simulink model "mariner_sim"  (R2018b)
settings: Solver=VariableStepAuto  StartTime=0.0  StopTime=10  RelTol=1e-3
libraries: simulink x1
settings Model: Creator=manzand  LastModifiedBy=manzand

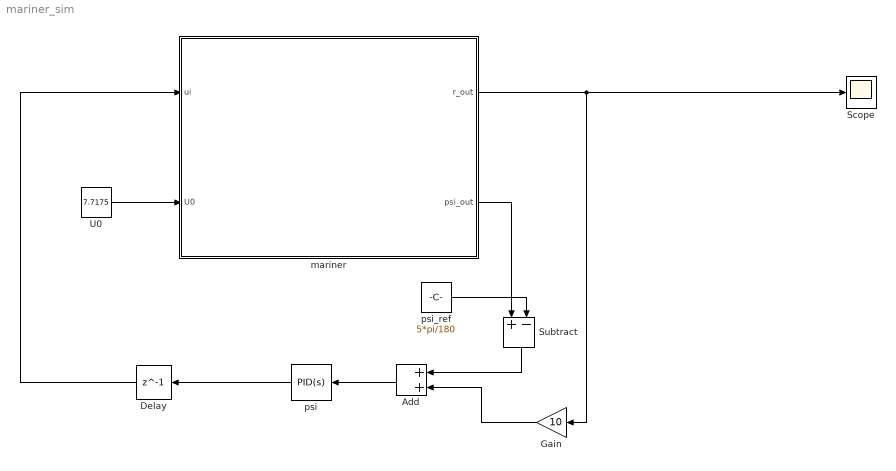
== system mariner_sim ==
  Add : Sum
  Delay : Delay  DelayLength=1  InitialCondition=0
  Gain : Gain  Gain=10
  Scope : Scope
  Subtract : Sum  Inputs=+-
  U0 : Constant  Value=7.7175
  mariner : Stateflow chart  TreatAsAtomicUnit=on
  psi : simulink/Continuous/PID Controller  Controller=PID  Form=Parallel  TimeDomain=Continuous-time  SampleTime=-1  IntegratorMethod=Forward Euler  FilterMethod=Forward Euler  ControllerParametersSource=internal  P=-1  I=0  D=0  UseFilter=on  N=100  TunerSelectOption=Transfer Function Based (PID Tuner App)  InitialConditionSource=internal  InitialConditionForIntegrator=0  InitialConditionForFilter=0  DifferentiatorICPrevScaledInput=0  ExternalReset=none  TrackingMode=off  Kt=1  LimitOutput=off  UpperSaturationLimit=inf  LowerSaturationLimit=-inf  LinearizeAsGain=on  AntiWindupMode=none  Kb=1  POutMin=[]  POutMax=[]  IOutMin=[]  IOutMax=[]  DOutMin=[]  DOutMax=[]  NOutMin=[]  NOutMax=[]  SumOutMin=[]  SumOutMax=[]  SaturationOutMin=[]  SaturationOutMax=[]  PParamMin=[]  PParamMax=[]  IParamMin=[]  IParamMax=[]  DParamMin=[]  DParamMax=[]  NParamMin=[]  NParamMax=[]  KbParamMin=[]  KbParamMax=[]  KtParamMin=[]  KtParamMax=[]  KbOutMin=[]  KbOutMax=[]  KtOutMin=[]  KtOutMax=[]  IntegratorOutMin=[]  IntegratorOutMax=[]  FilterOutMin=[]  FilterOutMax=[]  SumI1OutMin=[]  SumI1OutMax=[]  SumI2OutMin=[]  SumI2OutMax=[]  SumI3OutMin=[]  SumI3OutMax=[]  SumI4OutMin=[]  SumI4OutMax=[]  SumDOutMin=[]  SumDOutMax=[]  DifferentiatorOutMin=[]  DifferentiatorOutMax=[]  FilterDiffOutCoefMin=[]  FilterDiffOutCoefMax=[]  ReciprocalOutMin=[]  ReciprocalOutMax=[]  SumDenOutMin=[]  SumDenOutMax=[]  SumNumOutMin=[]  SumNumOutMax=[]  DivideOutMin=[]  DivideOutMax=[]  IntegratorContinuousStateAttributes=''  IntegratorStateMustResolveToSignalObject=off  IntegratorRTWStateStorageClass=Auto  FilterContinuousStateAttributes=''  FilterStateMustResolveToSignalObject=off  FilterRTWStateStorageClass=Auto  ParallelPVariant=InternalParameters  IdealPVariant=Disabled  IVariant=InternalParameters  DVariant=InternalParameters  IntegratorVariant=Continuous  SatVariant=Disabled  AWVariant=Passthrough  PCopyVariant=Disabled  TRVariant=Disabled  FdbkBlocksVariant=Forward  IdealPFdbkVariant=Disabled  SatFdbkVariant=Disabled  DerivativeFilterVariant=ContFilter  NVariant=InternalParameters  NCopyVariant=Disabled  FilterICVariant=InternalICsFilter  IntegratorICVariant=InternalICs  ExternalResetVariant=Disabled  TRSumVariant=Passthrough  SumFdbkVariant=Disabled  SumVariant=Sum_PID
  psi_ref : Constant  Value=5*pi/180
  wires:
  U0/1 -> mariner/2(U0)
  mariner/1(r_out) -> Scope/1, Gain/1
  mariner/2(psi_out) -> Subtract/1
  psi_ref/1 -> Subtract/2
  Subtract/1 -> Add/1
  Gain/1 -> Add/2
  Add/1 -> psi/1
  psi/1 -> Delay/1
  Delay/1 -> mariner/1(ui)

== stateflow chart mariner_sim/mariner ==
  settings: updateMethod=CONTINUOUS
  state mariner
    %% initialize values when entry
    en:
    L = 160.93;
    m = 798*10^-5;
    xG = -0.023;
    Iz = 39.2*10^-5;
    Xudot =  -42e-5;  Yvdot =  -748e-5;  Nvdot = 4.646e-5;
    Xu  = -184e-5;   Yrdot =-9.354e-5;   Nrdot = -43.8e-5;
    Xuu = -110e-5;   Yv = -1160e-5;   Nv =  -264e-5;
    Xuuu = -215e-5;   Yr =  -499e-5;   Nr =  -166e-5;
    Xvv = -899e-5;   Yvvv = -8078e-5;   Nvvv =  1636e-5;
    Xrr =   18e-5;   Yvvr = 15356e-5;   Nvvr = -5483e-5;
    Xdd =  -95e-5;   Yvu = -1160e-5;   Nvu =  -264e-5;
    Xudd = -190e-5;   Yru =  -499e-5;   Nru =  -166e-5;
    Xrv =  798e-5;   Yd  =   278e-5;   Nd =  -139e-5;
    Xvd =   93e-5;   Yddd  =   -90e-5;   Nddd =    45e-5;
    Xuvd =   93e-5;   Yud = 556e-5;   Nud =  -278e-5;
    Yuud =   278e-5;   Nuud  =  -139e-5;
    Yvdd  =    -4e-5;   Nvdd  = 13e-5;
    Yvvd  =  1190e-5;   Nvvd  = -489e-5;
    Y0 = -4e-5;   N0 =  3e-5;
    Y0u  =  -8e-5;   N0u = 6e-5;
    Y0uu =  -4e-5;   N0uu  =  3e-5;
    m11 = 798*10^-5 - (-42e-5);
    m22 = 798*10^-5 - ( -748e-5);
    m23 = 798*10^-5 * -0.023 - (-9.354e-5);
    m32 = 798*10^-5 * -0.023 - 4.646e-5;
    m33 = 39.2*10^-5 -  (-43.8e-5);
    %detM22 = m22*m33-m23*m32;
    %detM22 = ((798*10^-5 - ( -748e-5))*(39.2*10^-5 -  (-43.8e-5)) - (798*10^-5 * -0.023 - (-9.354e-5))*(798*10^-5 * -0.023 - 4.646e-5));
    delta_max = 40;
    Ddelta_max = 5;
    % u
    %Executing updates of system during simulation
    du:
    %delta_c = min(max(-ui,-delta_max*pi/180),delta_max*pi/180) ;
    %U = (sqrt((ui + u)^2 + v^2));
    %delta_do = (-ui - delta);
    %X = Xu*u/(sqrt((ui + u)^2 + v^2)) + Xuu*(u/(sqrt((ui + u)^2 + v^2)))^2 + Xuuu*(u/(sqrt((ui + u)^2 + v^2)))^3 + Xvv*(v/(sqrt((ui + u)^2 + v^2)))^2 + Xrr*(r*L/(sqrt((ui + u)^2 + v^2)))^2 + Xrv*(r*L/(sqrt((ui + u)^2 + v^2)))*(v/(sqrt((ui + u)^2 + v^2))) + Xdd*delta^2 +Xudd*(u/(sqrt((ui + u)^2 + v^2)))*delta^2 + Xvd*(v/(sqrt((ui + u)^2 + v^2)))*delta + Xuvd*(u/(sqrt((ui + u)^2 + v^2)))*(v/(sqrt((ui + u)^2 + v^2)))*delta;
    %Y = Yv*v + Yr*r + Yvvv*v^3 + Yvvr*v^2*r + Yvu*v*u + Yru*r*u + Yd*delta + Yddd*delta^3 + Yud*u*delta + Yuud*u^2*delta + Yvdd*v*delta^2 + Yvvd*v^2*delta + (Y0 + Y0u*u + Y0uu*u^2);
    %N = Nv*v + Nr*r + Nvvv*v^3 + Nvvr*v^2*r + Nvu*v*u + Nru*r*u + Nd*delta + Nddd*delta^3 + Nud*u*delta + Nuud*u^2*delta + Nvdd*v*delta^2 + Nvvd*v^2*delta + (N0 + N0u*u + N0uu*u^2);
    u_dot = (Xu*(u/(sqrt((ui + u)^2 + v^2))) + Xuu*(u/(sqrt((ui + u)^2 + v^2)))^2 + Xuuu*(u/(sqrt((ui + u)^2 + v^2)))^3 + Xvv*(v/(sqrt((ui + u)^2 + v^2)))^2 + Xrr*(r*L/(sqrt((ui + u)^2 + v^2)))^2 + Xrv*(r*L/(sqrt((ui + u)^2 + v^2)))*(v/(sqrt((ui + u)^2 + v^2))) + Xdd*delta^2 +Xudd*(u/(sqrt((ui + u)^2 + v^2)))*delta^2 + Xvd*(v/(sqrt((ui + u)^2 + v^2)))*delta + Xuvd*(u/(sqrt((ui + u)^2 + v^2)))*(v/(sqrt((ui + u)^2 + v^2)))*delta)*((sqrt((ui + u)^2 + v^2))^2 /L)/(798*10^-5 - (-42e-5));
    v_dot =  -(-(39.2*10^-5 -  (-43.8e-5))*(Yv*(v/(sqrt((ui + u)^2 + v^2))) + Yr*(r*L/(sqrt((ui + u)^2 + v^2))) + Yvvv*(v/(sqrt((ui + u)^2 + v^2)))^3 + Yvvr*(v/(sqrt((ui + u)^2 + v^2)))^2 * (r*L/(sqrt((ui + u)^2 + v^2))) + Yvu*(v/(sqrt((ui + u)^2 + v^2)))*(u/(sqrt((ui + u)^2 + v^2))) + Yru*(r*L/(sqrt((ui + u)^2 + v^2)))*(u/(sqrt((ui + u)^2 + v^2))) + Yd*delta + Yddd*delta^3 + Yud*(u/(sqrt((ui + u)^2 + v^2)))*delta + Yuud*(u/(sqrt((ui + u)^2 + v^2)))^2*delta + Yvdd*(v/(sqrt((ui + u)^2 + v^2)))*delta^2 + Yvvd*(v/(sqrt((ui + u)^2 + v^2)))^2*delta + (Y0 + Y0u*(u/(sqrt((ui + u)^2 + v^2))) + Y0uu*(u/(sqrt((ui + u)^2 + v^2)))^2))+(798*10^-5 * -0.023 - (-9.354e-5))*(Nv*(v/(sqrt((ui + u)^2 + v^2))) + Nr*(r*L/(sqrt((ui + u)^2 + v^2))) + Nvvv*(v/(sqrt((ui + u)^2 + v^2)))^3 + Nvvr*(v/(sqrt((ui + u)^2 + v^2)))^2*(r*L/(sqrt((ui + u)^2 + v^2))) + Nvu*(v/(sqrt((ui + u)^2 + v^2)))*(u/(sqrt((ui + u)^2 + v^2))) + Nru*(r*L/(sqrt((ui + u)^2 + v^2)))*(u/(sqrt((ui + u)^2 + v^2))) + Nd*delta + Nddd*delta^3 + Nud*(u/(sqrt((ui + u)^2 + v^2)))*delta + Nuud*(u/(sqrt((ui + u)^2 + v^2)))^2*delta + Nvdd*(v/(sqrt((ui + u)^2 + v^2)))*delta^2 + Nvvd*v^2*delta + (N0 + N0u*u + N0uu*u^2)))*((sqrt((ui + u)^2 + v^2))^2/L)/((798*10^-5 - ( -748e-5))*(39.2*10^-5 -  (-43.8e-5)) - (798*10^-5 * -0.023 - (-9.354e-5))*(798*10^-5 * -0.023 - 4.646e-5)) ;
    r_dot = (-(798*10^-5 * -0.023 - 4.646e-5)*(Yv*(v/(sqrt((ui + u)^2 + v^2))) + Yr*(r*L/(sqrt((ui + u)^2 + v^2))) + Yvvv*(v/(sqrt((ui + u)^2 + v^2)))^3 + Yvvr*(v/(sqrt((ui + u)^2 + v^2)))^2*(r*L/(sqrt((ui + u)^2 + v^2))) + Yvu*(v/(sqrt((ui + u)^2 + v^2)))*(u/(sqrt((ui + u)^2 + v^2))) + Yru*(r*L/(sqrt((ui + u)^2 + v^2)))*(u/(sqrt((ui + u)^2 + v^2))) + Yd*delta + Yddd*delta^3 + Yud*(u/(sqrt((ui + u)^2 + v^2)))*delta + Yuud*(u/(sqrt((ui + u)^2 + v^2)))^2*delta + Yvdd*(v/(sqrt((ui + u)^2 + v^2)))*delta^2 + Yvvd*(v/(sqrt((ui + u)^2 + v^2)))^2*delta + (Y0 + Y0u*(u/(sqrt((ui + u)^2 + v^2))) + Y0uu*(u/(sqrt((ui + u)^2 + v^2)))^2))+(798*10^-5 - ( -748e-5))*(Nv*(v/(sqrt((ui + u)^2 + v^2))) + Nr*(r*L/(sqrt((ui + u)^2 + v^2))) + Nvvv*(v/(sqrt((ui + u)^2 + v^2)))^3 + Nvvr*(v/(sqrt((ui + u)^2 + v^2)))^2*(r*L/(sqrt((ui + u)^2 + v^2))) + Nvu*(v/(sqrt((ui + u)^2 + v^2)))*(u/(sqrt((ui + u)^2 + v^2))) + Nru*(r*L/(sqrt((ui + u)^2 + v^2)))*(u/(sqrt((ui + u)^2 + v^2))) + Nd*delta + Nddd*delta^3 + Nud*(u/(sqrt((ui + u)^2 + v^2)))*delta + Nuud*(u/(sqrt((ui + u)^2 + v^2)))^2*delta + Nvdd*(v/(sqrt((ui + u)^2 + v^2)))*delta^2 + Nvvd*(v/(sqrt((ui + u)^2 + v^2)))^2*delta + (N0 + N0u*(u/(sqrt((ui + u)^2 + v^2))) + N0uu*(u/(sqrt((ui + u)^2 + v^2)))^2)))*((sqrt((ui + u)^2 + v^2))^2/L^2)/((798*10^-5 - ( -748e-5))*(39.2*10^-5 -  (-43.8e-5)) - (798*10^-5 * -0.023 - (-9.354e-5))*(798*10^-5 * -0.023 - 4.646e-5)) ;
    x_dot = (cos(psi)*(U0/(sqrt((ui + u)^2 + v^2))+(u/(sqrt((ui + u)^2 + v^2))))-sin(psi)*(v/(sqrt((ui + u)^2 + v^2))))*(sqrt((ui + u)^2 + v^2)) ;
    y_dot = (sin(psi)*(U0/(sqrt((ui + u)^2 + v^2))+(u/(sqrt((ui + u)^2 + v^2))))+cos(psi)*(v/(sqrt((ui + u)^2 + v^2))))*(sqrt((ui + u)^2 + v^2)) ;
    psi_dot = (r*L/(sqrt((ui + u)^2 + v^2)))*((sqrt((ui + u)^2 + v^2))/L);
    delta_dot = min(max(((min(max(-ui,-delta_max*pi/180),delta_max*pi/180)) - delta),-Ddelta_max*pi/180),Ddelta_max*pi/180) ;
    %% OUTPUTS
    r_out = r;
    psi_out = psi;
  (default) -> mariner : {u = 0.01;
      | v = 0.01;
      | r = 0.01;
      | x = 0.01;
      | y = 0.01;
      | psi = 0.01;
      | delta = 0.01;}
  data: u local; ui input; v local; Nvdot local double; Iz local double; L local double; Yvdot local double; xG local double; m local double; Xudot local double; Xuu local double; Yv local double; Xuuu local double; Nrdot local double; Nv local double; Yr local double; Yrdot local double; Xu local double; Nr local double; Xrr local double; Xdd local double; Yvvv local double; Yvu local double; Nvvv local double; Yvvr local double; Nvvr local double; Xvv local double; Xvd local double; Yru local double; Nd local double; Nvu local double; Xudd local double; Nru local double; Yd local double; Xrv local double; Nvdd local double; Yud local double; Yuud local double; Xuvd local double; Yvdd local double; Nud local double; Nuud local double; Yddd local double; Nddd local double; Y0uu local double; N0uu local double; N0 local double; N0u local double; Y0 local double; Yvvd local double; Nvvd local double; Y0u local double; m11 local double; m32 local double; m22 local double; m23 local double; m33 local double; U0 input; r_out output; r local; psi local; x local; y local; delta local; psi_out output double; Ddelta_max local double; delta_max local double; N local double
  data u settings: updateMethod=SF_CONTINUOUS_TIME_DATA
  data v settings: updateMethod=SF_CONTINUOUS_TIME_DATA
  data r settings: updateMethod=SF_CONTINUOUS_TIME_DATA
  data psi settings: updateMethod=SF_CONTINUOUS_TIME_DATA
  data x settings: updateMethod=SF_CONTINUOUS_TIME_DATA
  data y settings: updateMethod=SF_CONTINUOUS_TIME_DATA
  data delta settings: updateMethod=SF_CONTINUOUS_TIME_DATA
